simulink model "lab2_fixp"  (R2022a)
settings: Solver=VariableStepAuto  StartTime=0.0  StopTime=10.0  RelTol=1e-3
settings Model: Creator=user  LastModifiedBy=user

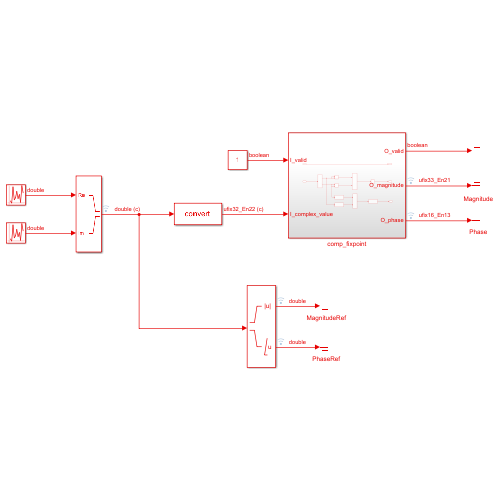
[thumbnail: Simulink's stored preview of the top-level diagram]
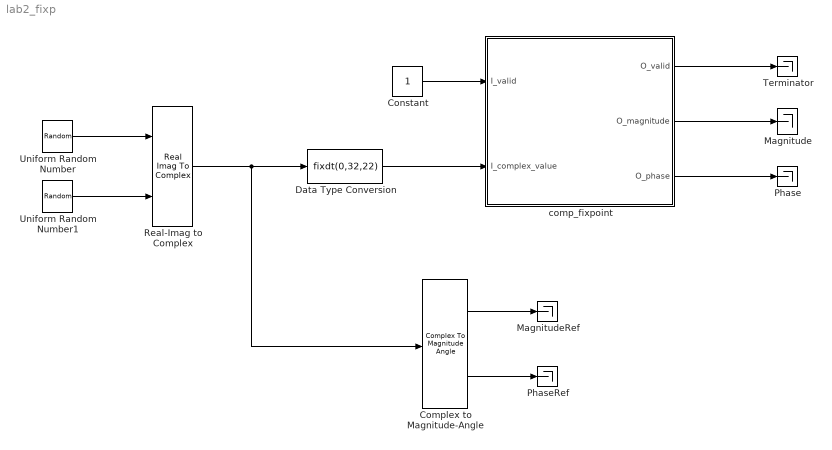
== system lab2_fixp ==
  Complex to Magnitude-Angle : ComplexToMagnitudeAngle
  Constant : Constant  OutDataTypeStr=boolean  SampleTime=1
  Data Type Conversion : DataTypeConversion  OutDataTypeStr=fixdt(0,32,22)  RndMeth=Round
  Magnitude : Terminator
  MagnitudeRef : Terminator
  Phase : Terminator
  PhaseRef : Terminator
  Real-Imag to Complex : RealImagToComplex
  Terminator : Terminator
  Uniform Random Number : UniformRandomNumber  Minimum=0  Maximum=1023.99999976158142089844  Seed=10  SampleTime=1
  Uniform Random Number1 : UniformRandomNumber  Minimum=0  Maximum=1023.99999976158142089844  Seed=11  SampleTime=1
  comp_fixpoint : Subsystem
  wires:
  Uniform Random Number1/1 -> Real-Imag to Complex/2
  Uniform Random Number/1 -> Real-Imag to Complex/1
  Real-Imag to Complex/1 -> Complex to Magnitude-Angle/1, Data Type Conversion/1
  Constant/1 -> comp_fixpoint/1(I_valid)
  comp_fixpoint/1(O_valid) -> Terminator/1
  Data Type Conversion/1 -> comp_fixpoint/2(I_complex_value)
  comp_fixpoint/3(O_phase) -> Phase/1
  comp_fixpoint/2(O_magnitude) -> Magnitude/1
  Complex to Magnitude-Angle/1 -> MagnitudeRef/1
  Complex to Magnitude-Angle/2 -> PhaseRef/1

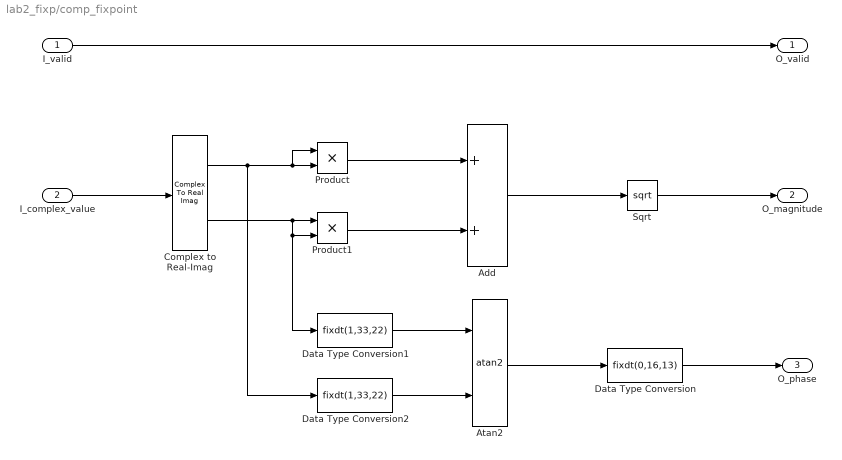
== system lab2_fixp/comp_fixpoint ==
  I_valid : Inport
  I_complex_value : Inport  Port=2
  Add : Sum
  Atan2 : Trigonometry  Operator=atan2  ApproximationMethod=CORDIC  NumberOfIterations=20
  Complex to Real-Imag : ComplexToRealImag
  Data Type Conversion : DataTypeConversion  OutDataTypeStr=fixdt(0,16,13)  RndMeth=Round  SaturateOnIntegerOverflow=off
  Data Type Conversion1 : DataTypeConversion  OutDataTypeStr=fixdt(1,33,22)  SaturateOnIntegerOverflow=off  RndMeth=Floor
  Data Type Conversion2 : DataTypeConversion  OutDataTypeStr=fixdt(1,33,22)  SaturateOnIntegerOverflow=off  RndMeth=Floor
  Product : Product
  Product1 : Product
  Sqrt : Sqrt  OutDataTypeStr=fixdt(0,33,21)
  O_valid : Outport
  O_magnitude : Outport  Port=2
  O_phase : Outport  Port=3
  wires:
  I_valid/1 -> O_valid/1
  I_complex_value/1 -> Complex to Real-Imag/1
  Complex to Real-Imag/1 -> Data Type Conversion2/1, Product/1, Product/2
  Complex to Real-Imag/2 -> Data Type Conversion1/1, Product1/2, Product1/1
  Product1/1 -> Add/2
  Product/1 -> Add/1
  Add/1 -> Sqrt/1
  Sqrt/1 -> O_magnitude/1
  Atan2/1 -> Data Type Conversion/1
  Data Type Conversion/1 -> O_phase/1
  Data Type Conversion1/1 -> Atan2/1
  Data Type Conversion2/1 -> Atan2/2
